simulink model "CSE_Dimapasoc_Cassius_BlockDiagramAlgebra_No1_Simulink.m"  (R2023b)
settings: Solver=VariableStepAuto  StartTime=0.0  StopTime=10.0  RelTol=1e-3
settings Model: Creator=nicole  LastModifiedBy=nicole

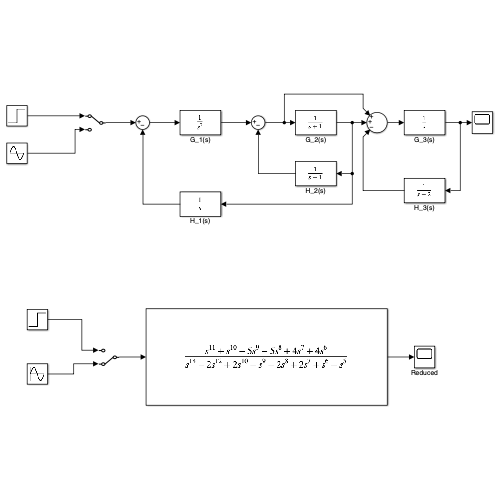
[thumbnail: Simulink's stored preview of the top-level diagram]
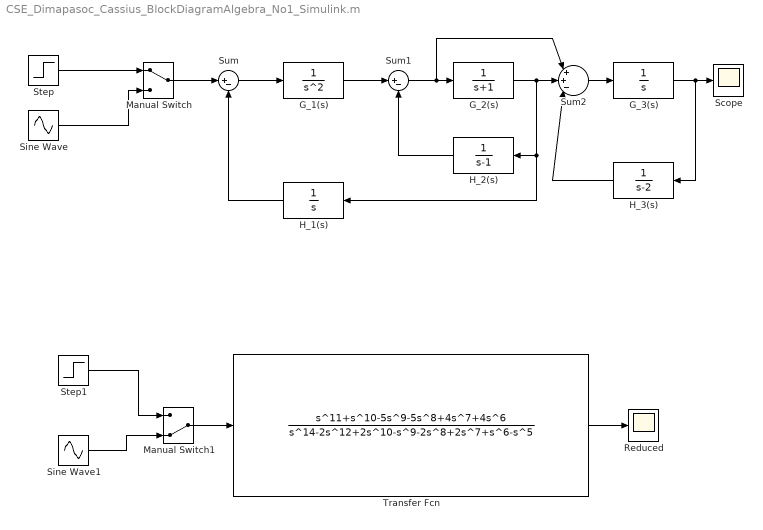
== system CSE_Dimapasoc_Cassius_BlockDiagramAlgebra_No1_Simulink.m ==
  G_1(s) : TransferFcn  Numerator=[0 0 1]  Denominator=[1 0 0]
  G_2(s) : TransferFcn  Numerator=[0 0 1]  Denominator=[1 1]
  G_3(s) : TransferFcn  Numerator=[0 1]  Denominator=[1 0]
  H_1(s) : TransferFcn  Numerator=[0 1]  Denominator=[1 0]
  H_2(s) : TransferFcn  Numerator=[0 1]  Denominator=[1 -1]
  H_3(s) : TransferFcn  Numerator=[0 1]  Denominator=[1 -2]
  Manual Switch : ManualSwitch
  Manual Switch1 : ManualSwitch  CurrentSetting=0
  Reduced : Scope
  Scope : Scope
  Sine Wave : Sin  SampleTime=0
  Sine Wave1 : Sin  SampleTime=0
  Step : Step  Time=0  SampleTime=0
  Step1 : Step  SampleTime=0
  Sum : Sum  Inputs=|+-
  Sum1 : Sum  Inputs=|+-
  Sum2 : Sum  Inputs=|++-|
  Transfer Fcn : TransferFcn  Numerator=[1 1 -5 -5 4 4 0 0 0 0 0 0]  Denominator=[1 0 -2 0 2 -1 -2 2 1 -1 0 0 0 0 0]  ParameterTunability=Optimized
  wires:
  G_1(s)/1 -> Sum1/1
  Sum/1 -> G_1(s)/1
  Sum2/1 -> G_3(s)/1
  G_2(s)/1 -> H_1(s)/1, H_2(s)/1, Sum2/2
  Sum1/1 -> Sum2/1, G_2(s)/1
  G_3(s)/1 -> H_3(s)/1, Scope/1
  H_1(s)/1 -> Sum/2
  H_2(s)/1 -> Sum1/2
  H_3(s)/1 -> Sum2/3
  Transfer Fcn/1 -> Reduced/1
  Manual Switch/1 -> Sum/1
  Step/1 -> Manual Switch/1
  Sine Wave/1 -> Manual Switch/2
  Step1/1 -> Manual Switch1/1
  Manual Switch1/1 -> Transfer Fcn/1
  Sine Wave1/1 -> Manual Switch1/2
